simulink model "trial"  (R2021a)
settings: Solver=VariableStepAuto  StartTime=0.0  StopTime=10.0  RelTol=1e-3
settings Model: Creator=USER  LastModifiedBy=USER

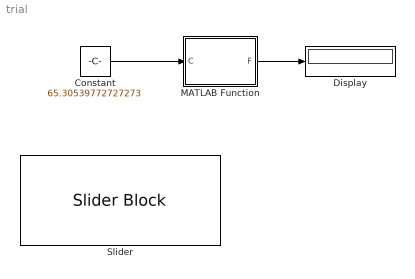
== system trial ==
  Constant : Constant  Value=65.30539772727273
  Display : Display
  MATLAB Function : MATLAB Function  TreatAsAtomicUnit=on
  Slider : SliderBlock
  wires:
  Constant/1 -> MATLAB Function/1(C)
  MATLAB Function/1(F) -> Display/1

== matlab function trial/MATLAB Function ==
  data: C input; F output
function F = conv_temp(C)

F = (C+5)/2;
